simulink model "testmodel"  (R2024b)
settings: Solver=ode23t  StartTime=0.0  StopTime=10  FixedStep=0.0001  MaxStep=0.2  MinStep=0.0001  RelTol=1e-3
model workspace (MAT data in the model file):
  L = 0.57
  La = 0.000279
  Ra = 0.288
  ahead = 0.75
  d = 0.74
  maxrpm = 6000
  pathx : Simulink.Parameter (value not decoded)
  pathy : Simulink.Parameter (value not decoded)
  rover_accel = 0.5
  roveracc = 0.5
  stepangle = 1.8
  w_r = 0.1
  wheelbase = 1
symbols that are objects in the model workspace (value not decoded): pathx, pathy
undefined symbols (not defined in the file): Discrete, Time
libraries: fl_lib x100, nesl_utility x53, ee_lib x15, slpidlib x5, ctrlSharedLib x3, robotalgslib x1, simulink x1
(part 2 of 3)

== system testmodel/control ==
  pos : Inport
  alpha : Inport  Port=2
  R : Inport  Port=3
  goal : Inport  Port=4
  actspeed : Inport  Port=5
  actang : Inport  Port=6
  Constant1 : Constant  Value=d*0.5
  Constant7 : Constant  Value=L
  Mux1 : Mux  Inputs=6
  PID Controller : slpidlib/PID Controller  Controller=PID  Form=Parallel  TimeDomain=Discrete-time  UseExternalTs=off  SampleTime=-1  IntegratorMethod=Forward Euler  FilterMethod=Forward Euler  ControllerParametersSource=internal  P=54.7409706092039  I=0.00122680114575866  UseKiTs=on  D=0.198895104349163  UseExternalDerivativeSource=off  N=8689.11352061538  UseFilter=on  TunerSelectOption=Transfer Function Based (PID Tuner App)  InitialConditionSource=internal  InitialConditionForIntegrator=0  InitialConditionForFilter=0  DifferentiatorICPrevScaledInput=0  ExternalReset=none  TrackingMode=off  Kt=1  LimitOutput=off  SatLimitsSource=internal  UpperSaturationLimit=inf  LowerSaturationLimit=-inf  LinearizeAsGain=on  AntiWindupMode=none  Kb=1  LimitIntegrator=off  UpperIntegratorSaturationLimit=inf  LowerIntegratorSaturationLimit=-inf  POutMin=[]  POutMax=[]  IOutMin=[]  IOutMax=[]  DOutMin=[]  DOutMax=[]  NOutMin=[]  NOutMax=[]  SumOutMin=[]  SumOutMax=[]  SaturationOutMin=[]  SaturationOutMax=[]  PParamMin=[]  PParamMax=[]  IParamMin=[]  IParamMax=[]  DParamMin=[]  DParamMax=[]  NParamMin=[]  NParamMax=[]  KbParamMin=[]  KbParamMax=[]  KtParamMin=[]  KtParamMax=[]  KbOutMin=[]  KbOutMax=[]  KtOutMin=[]  KtOutMax=[]  IntegratorOutMin=[]  IntegratorOutMax=[]  FilterOutMin=[]  FilterOutMax=[]  SumI1OutMin=[]  SumI1OutMax=[]  SumI2OutMin=[]  SumI2OutMax=[]  SumI3OutMin=[]  SumI3OutMax=[]  SumI4OutMin=[]  SumI4OutMax=[]  SumDOutMin=[]  SumDOutMax=[]  DifferentiatorOutMin=[]  DifferentiatorOutMax=[]  FilterDiffOutCoefMin=[]  FilterDiffOutCoefMax=[]  ReciprocalOutMin=[]  ReciprocalOutMax=[]  SumDenOutMin=[]  SumDenOutMax=[]  SumNumOutMin=[]  SumNumOutMax=[]  DivideOutMin=[]  DivideOutMax=[]  UdiffTsProdOutMin=[]  UdiffTsProdOutMax=[]  NTsProdOutMin=[]  NTsProdOutMax=[]  UintegralTsProdOutMin=[]  UintegralTsProdOutMax=[]  UngainTsProdOutMin=[]  UngainTsProdOutMax=[]  ClampingZeroOutDataTypeStr=Inherit: Inherit via back propagation  ClampingZeroOutMin=[]  ClampingZeroOutMax=[]  FilterDenConstantOutDataTypeStr=Inherit: Inherit via back propagation  FilterDenConstantOutMin=[]  FilterDenConstantOutMax=[]  PCopyOutDataTypeStr=Inherit: Inherit via back propagation  PCopyOutMin=[]  PCopyOutMax=[]  NCopyOutDataTypeStr=Inherit: Inherit via back propagation  NCopyOutMin=[]  NCopyOutMax=[]  IntegratorContinuousStateAttributes=''  IntegratorStateMustResolveToSignalObject=off  IntegratorRTWStateStorageClass=Auto  FilterContinuousStateAttributes=''  FilterStateMustResolveToSignalObject=off  FilterRTWStateStorageClass=Auto  ParallelPVariant=InternalParameters  IdealPVariant=Disabled  IVariant=InternalParameters  DVariant=InternalParameters  IntegratorVariant=Discrete  SatVariant=Disabled  AWVariant=Passthrough  PCopyVariant=Disabled  TRVariant=Disabled  FdbkBlocksVariant=Forward  IdealPFdbkVariant=Disabled  SatFdbkVariant=Disabled  DerivativeFilterVariant=ForwardEulerFilter  NVariant=InternalParameters  NCopyVariant=Disabled  FilterICVariant=InternalICsFilter  IntegratorICVariant=InternalICs  ExternalResetVariant=Disabled  TRSumVariant=Passthrough  SumFdbkVariant=Disabled  SumVariant=Sum_PID  TsampFilterVariant=InternalTs  TsampNgainVariant=Passthrough  TsampIntegralVariant=Disabled_SignalSpec  ExternalSaturationOutDataTypeStr=Inherit: Same as second input  DerivativeSourceVariant=ErrorSignal  PreIntVariant=InternalPreInt
  Saturation : Saturate  UpperLimit=24  LowerLimit=-24
  Subsystem1 : Subsystem
  Sum : Sum  Inputs=|+-
  Sum1 : Sum  Inputs=|+-
  Unit Delay : UnitDelay  SampleTime=-1  HasFrameUpgradeWarning=on
  desspeed : Outport
  control : Outport  Port=2
  desang : Outport  Port=3
  angerror : Outport  Port=4
  wires:
  Subsystem1/2(wheel_speed_LM) -> Mux1/2
  Mux1/1 -> Sum/1, desspeed/1
  Subsystem1/3(wheel_speed_LB) -> Mux1/3
  actspeed/1 -> Sum/2
  PID Controller/1 -> Unit Delay/1
  Subsystem1/4(wheel_speed_RF) -> Mux1/4
  Sum/1 -> PID Controller/1
  Subsystem1/6(wheel_speed_RB) -> Mux1/6
  Subsystem1/1(wheel_speed_LF) -> Mux1/1
  Unit Delay/1 -> Saturation/1
  Subsystem1/5(wheel_speed_RM) -> Mux1/5
  alpha/1 -> Subsystem1/1(alpha)
  Constant1/1 -> Subsystem1/3(d)
  Constant7/1 -> Subsystem1/2("L ")
  Saturation/1 -> control/1
  R/1 -> Subsystem1/4("R ")
  pos/1 -> Subsystem1/5(pos)
  goal/1 -> Subsystem1/6(goal)
  Subsystem1/7(desang) -> Sum1/1, desang/1
  actang/1 -> Sum1/2
  Sum1/1 -> angerror/1

== system testmodel/driver ==
  bodyangle : Inport
  gpspos : Inport  Port=2
  encoderpos : Inport  Port=3
  angvwheels : Inport  Port=4
  ref : Inport  Port=5
  bodyangle1 : Inport  Port=6
  gpspos1 : Inport  Port=7
  code : Subsystem
  sim : Subsystem
  controlsignal : Outport
  wires:
  bodyangle/1 -> code/1(bodyangle)
  gpspos/1 -> code/2(gpspos)
  encoderpos/1 -> code/3(encoderpos)
  angvwheels/1 -> code/4(angvwheels)
  ref/1 -> code/5(ref)
  code/1(controlsignal) -> controlsignal/1
  bodyangle1/1 -> sim/1(bodyangle1)
  gpspos1/1 -> sim/2(gpspos1)

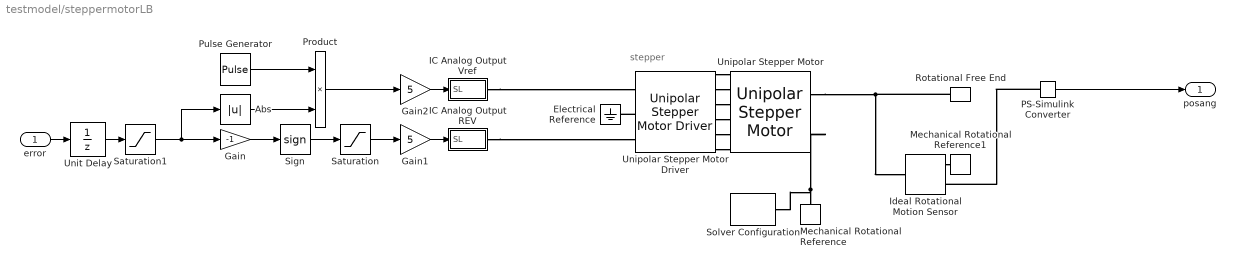
== system testmodel/steppermotorLB ==
  note: stepper
  error : Inport
  Abs : Abs  SaturateOnIntegerOverflow=off
  Electrical Reference : fl_lib/Electrical/Electrical Elements/Electrical Reference
  Gain : Gain  Gain=-1
  Gain1 : Gain  Gain=5
  Gain2 : Gain  Gain=5
  IC Analog Output REV : Subsystem
  IC Analog Output Vref : Subsystem
  Ideal Rotational Motion Sensor : fl_lib/Mechanical/Mechanical Sensors/Ideal Rotational Motion Sensor  reference=foundation.enum.MeasurementReference.difference  acceleration_port=false  velocity_port=false  position_port=true  wrap_angle=false  offset=0 rad
      settings: InternalSimscapePortConfiguration="{\"Bottom\":[],\"Left\":[{\"id\":\"R\",\"label\":\"R\",\"type\":\"foundation.mechanical.rotational.rotational\"}],\"Right\":[{\"id\":\"C\",\"label\":\"C\",\"type\":\"foundation.mechanical.rotational.rotational\"},{\"id\":\"A\",\"label\":\"A\",\"type\":\"output\"}],\"Top\":[]}"
  Mechanical Rotational Reference : fl_lib/Mechanical/Rotational Elements/Mechanical Rotational Reference
  Mechanical Rotational Reference1 : fl_lib/Mechanical/Rotational Elements/Mechanical Rotational Reference
  PS-Simulink Converter : nesl_utility/PS-Simulink Converter  PhysicalDomain=network_engine_domain  SubClassName=ps_output  LeftPortType=input  RightPortType=output  PseudoPeriodic=off  Frequencies=[]  VectorFormat=inherit  Unit=inherit  AffineConversion=off
  Product : Product
  Pulse Generator : DiscretePulseGenerator  Period=10  SampleTime=0.0001
  Rotational Free End : fl_lib/Mechanical/Rotational Elements/Rotational Free End  w_specify=off  w_priority=None  w=0 rad/s  w_nominal_specify=off  w_nominal_value=1  w_nominal_unit=rad/s
  Saturation : Saturate  UpperLimit=1  LowerLimit=0
  Saturation1 : Saturate  UpperLimit=1  LowerLimit=-1
  Sign : Signum
  Solver Configuration : nesl_utility/Solver Configuration  PhysicalDomain=network_engine_domain  SubClassName=solver  LeftPortType=input  RightPortType=generic  Tones=[]  Harmonics=[]  SimulateNoise=off  Profile=off  UseLocalSampling=off  EnableSwitchedLinearOptims=on  FrequencyDomain=off  UseCCode=off  RelTol=0.001  AbsTol=0.001  MinStep=1e-09  ToWorkspace=off  RevertToSquareIcSolve=off  NumHomotopyIterations=100  PhasorMode=off  PhasorModeNumHarmonics=1  ConsistencySolver=NEWTON_XTOL_AFTER_FTOL  IndexReductionMethod=DerivativeReplacement  DoDC=off  ResidualTolerance=1e-09  ConsistencyTolSource=GLOBAL  ConsistencyAbsTol=0.001  ConsistencyRelTol=0.001  ConsistencyTolFactor=0.001  UseLocalSolver=on  LocalSolverChoice=NE_TRAPEZOIDAL_ADVANCER  ResolveIndetEquations=on  FunctionEvalNumThread=1  LocalSolverSampleTime=0.0001  DoFixedCost=off  MaxNonlinIter=3  MaxModeIter=2  ComputeImpulses=off  ImpulseIterations=2  LinearAlgebra=auto  LinearAlgebraNumThread=0  EquationFormulation=NE_TIME_EF  DelaysMemoryBudget=1024  AutomaticFiltering=on  FilteringTimeConstant=0.001  PartitionStorageMethod=AS_NEEDED  PartitionMemoryBudget=1024  PartitionMethod=ROBUST  MultibodyUseLocalSolver=off  MultibodyLocalSolverChoice=ODE1  MultibodyLocalSolverSampleTime=0.001
  Unipolar Stepper Motor : ee_lib/Electromechanical/Reluctance & Stepper/Unipolar Stepper Motor  step_or_av=ee.enum.electromech.simulationMode.stepping  Ra=0.9 Ohm  La=2.2 mH  k=0  Km=0.19 N*m/A  Td=0 N*m  Rm=inf Ohm  w_vec=[0, 1000, 3000] rpm  T_vec=[2, 2, 1] N*m  assert_if_slipping=ee.enum.assertAction.none  J_total=1e-4 kg*m^2  max_step_rate=10 Hz  Step=1.8 deg  J=3.6e-5 kg*m^2  B=8.0e-4 N*m*s/rad  speed0=0 rpm  theta0=0 deg  alpha=3.93e-3 1/K  Tmeas=25 degC  Tmeas2=125 degC  T_vec2=[1.7, 1.7, .85] N*m  half_stepping=ee.enum.electromech.steppingModeAveraged.fullStep  thermal_mass=100 J/K  initial_temperatures=[25, 25, 25, 25] degC  rotor_thermal_mass=50 J/K  rotor_initial_temperature=25 degC  Rm_percent_rotor=90
      settings: InternalSimscapePortConfiguration="{\"Bottom\":[],\"Left\":[{\"id\":\"pA\",\"label\":\"A+\",\"type\":\"foundation.electrical.electrical\"},{\"id\":\"cA\",\"label\":\"A0\",\"type\":\"foundation.electrical.electrical\"},{\"id\":\"nA\",\"label\":\"A-\",\"type\":\"foundation.electrical.electrical\"},{\"id\":\"pB\",\"label\":\"B+\",\"type\":\"foundation.electrical.electrical\"},{\"id\":\"cB\",\"label\":\"B0\",\"type\":\"foundation.electrical.electrical\"},{\"id\":\"nB\",\"label\":\"B-\",\"type\":\"foundation.electrical.electrical\"}],\"Right\":[{\"id\":\"R\",\"label\":\"R\",\"type\":\"foundation.mechanical.rotational.rotational\"},{\"id\":\"C\",\"label\":\"C\",\"type\":\"foundation.mechanical.rotational.rotational\"}],\"Top\":[]}"
  Unipolar Stepper Motor Driver : ee_lib/Electromechanical/Reluctance & Stepper/Unipolar Stepper Motor Driver  step_or_av=ee.enum.electromech.simulationMode.stepping  step_rate_per_volt=10 Hz/V  Venable=0.1 V  Vreverse=0.1 V  Vm=24 V  half_stepping=ee.enum.electromech.steppingModeAveraged.fullStep
      settings: InternalSimscapePortConfiguration="{\"Bottom\":[],\"Left\":[{\"id\":\"ENA\",\"label\":\"ENA\",\"type\":\"foundation.electrical.electrical\"},{\"id\":\"REF\",\"label\":\"REF\",\"type\":\"foundation.electrical.electrical\"},{\"id\":\"REV\",\"label\":\"REV\",\"type\":\"foundation.electrical.electrical\"}],\"Right\":[{\"id\":\"pA\",\"label\":\"A+\",\"type\":\"foundation.electrical.electrical\"},{\"id\":\"cA\",\"label\":\"A0\",\"type\":\"foundation.electrical.electrical\"},{\"id\":\"nA\",\"label\":\"A-\",\"type\":\"foundation.electrical.electrical\"},{\"id\":\"pB\",\"label\":\"B+\",\"type\":\"foundation.electrical.electrical\"},{\"id\":\"cB\",\"label\":\"B0\",\"type\":\"foundation.electrical.electrical\"},{\"id\":\"nB\",\"label\":\"B-\",\"type\":\"foundation.electrical.electrical\"}],\"Top\":[]}"
  Unit Delay : UnitDelay  SampleTime=-1  HasFrameUpgradeWarning=on
  posang : Outport
  wires:
  PS-Simulink Converter/1 -> posang/1
  Gain/1 -> Sign/1
  Sign/1 -> Saturation/1
  Pulse Generator/1 -> Product/1
  Saturation/1 -> Gain1/1
  Product/1 -> Gain2/1
  Gain2/1 -> IC Analog Output Vref/1(SL)
  Gain1/1 -> IC Analog Output REV/1(SL)
  Abs/1 -> Product/2
  Saturation1/1 -> Abs/1, Gain/1
  error/1 -> Unit Delay/1
  Unit Delay/1 -> Saturation1/1
  connections:
  Unipolar Stepper Motor Driver/RConn3 -- Unipolar Stepper Motor/LConn3
  Unipolar Stepper Motor Driver/RConn1 -- Unipolar Stepper Motor/LConn1
  Unipolar Stepper Motor Driver/RConn6 -- Unipolar Stepper Motor/LConn6
  Unipolar Stepper Motor Driver/RConn2 -- Unipolar Stepper Motor/LConn2
  Unipolar Stepper Motor Driver/RConn4 -- Unipolar Stepper Motor/LConn4
  Unipolar Stepper Motor Driver/RConn5 -- Unipolar Stepper Motor/LConn5
  Unipolar Stepper Motor/RConn1 -- Ideal Rotational Motion Sensor/LConn1 -- Rotational Free End/LConn1
  Unipolar Stepper Motor Driver/LConn2 -- Electrical Reference/LConn1
  PS-Simulink Converter/LConn1 -- Ideal Rotational Motion Sensor/RConn2
  Ideal Rotational Motion Sensor/RConn1 -- Mechanical Rotational Reference1/LConn1
  Mechanical Rotational Reference/LConn1 -- Unipolar Stepper Motor/RConn2 -- Solver Configuration/RConn1
  IC Analog Output Vref/RConn1 -- Unipolar Stepper Motor Driver/LConn1
  IC Analog Output REV/RConn1 -- Unipolar Stepper Motor Driver/LConn3

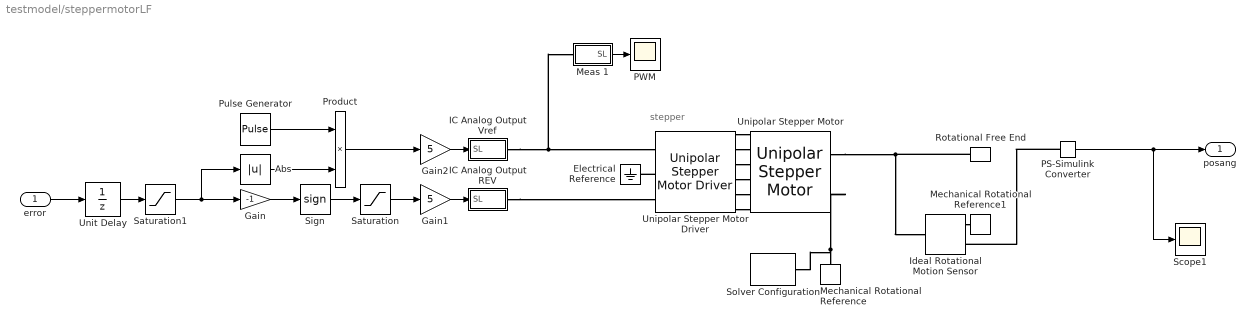
== system testmodel/steppermotorLF ==
  note: stepper
  error : Inport
  Abs : Abs  SaturateOnIntegerOverflow=off
  Electrical Reference : fl_lib/Electrical/Electrical Elements/Electrical Reference
  Gain : Gain  Gain=-1
  Gain1 : Gain  Gain=5
  Gain2 : Gain  Gain=5
  IC Analog Output REV : Subsystem
  IC Analog Output Vref : Subsystem
  Ideal Rotational Motion Sensor : fl_lib/Mechanical/Mechanical Sensors/Ideal Rotational Motion Sensor  reference=foundation.enum.MeasurementReference.difference  acceleration_port=false  velocity_port=false  position_port=true  wrap_angle=false  offset=0 rad
      settings: InternalSimscapePortConfiguration="{\"Bottom\":[],\"Left\":[{\"id\":\"R\",\"label\":\"R\",\"type\":\"foundation.mechanical.rotational.rotational\"}],\"Right\":[{\"id\":\"C\",\"label\":\"C\",\"type\":\"foundation.mechanical.rotational.rotational\"},{\"id\":\"A\",\"label\":\"A\",\"type\":\"output\"}],\"Top\":[]}"
  Meas 1 : Subsystem
  Mechanical Rotational Reference : fl_lib/Mechanical/Rotational Elements/Mechanical Rotational Reference
  Mechanical Rotational Reference1 : fl_lib/Mechanical/Rotational Elements/Mechanical Rotational Reference
  PS-Simulink Converter : nesl_utility/PS-Simulink Converter  PhysicalDomain=network_engine_domain  SubClassName=ps_output  LeftPortType=input  RightPortType=output  PseudoPeriodic=off  Frequencies=[]  VectorFormat=inherit  Unit=inherit  AffineConversion=off
  PWM : Scope
  Product : Product
  Pulse Generator : DiscretePulseGenerator  Period=10  SampleTime=0.0001
  Rotational Free End : fl_lib/Mechanical/Rotational Elements/Rotational Free End  w_specify=off  w_priority=None  w=0 rad/s  w_nominal_specify=off  w_nominal_value=1  w_nominal_unit=rad/s
  Saturation : Saturate  UpperLimit=1  LowerLimit=0
  Saturation1 : Saturate  UpperLimit=1  LowerLimit=-1
  Scope1 : Scope
  Sign : Signum
  Solver Configuration : nesl_utility/Solver Configuration  PhysicalDomain=network_engine_domain  SubClassName=solver  LeftPortType=input  RightPortType=generic  Tones=[]  Harmonics=[]  SimulateNoise=off  Profile=off  UseLocalSampling=off  EnableSwitchedLinearOptims=on  FrequencyDomain=off  UseCCode=off  RelTol=0.001  AbsTol=0.001  MinStep=1e-09  ToWorkspace=off  RevertToSquareIcSolve=off  NumHomotopyIterations=100  PhasorMode=off  PhasorModeNumHarmonics=1  ConsistencySolver=NEWTON_XTOL_AFTER_FTOL  IndexReductionMethod=DerivativeReplacement  DoDC=off  ResidualTolerance=1e-09  ConsistencyTolSource=GLOBAL  ConsistencyAbsTol=0.001  ConsistencyRelTol=0.001  ConsistencyTolFactor=0.001  UseLocalSolver=on  LocalSolverChoice=NE_TRAPEZOIDAL_ADVANCER  ResolveIndetEquations=on  FunctionEvalNumThread=1  LocalSolverSampleTime=0.0001  DoFixedCost=off  MaxNonlinIter=3  MaxModeIter=2  ComputeImpulses=off  ImpulseIterations=2  LinearAlgebra=auto  LinearAlgebraNumThread=0  EquationFormulation=NE_TIME_EF  DelaysMemoryBudget=1024  AutomaticFiltering=on  FilteringTimeConstant=0.001  PartitionStorageMethod=AS_NEEDED  PartitionMemoryBudget=1024  PartitionMethod=ROBUST  MultibodyUseLocalSolver=off  MultibodyLocalSolverChoice=ODE1  MultibodyLocalSolverSampleTime=0.001
  Unipolar Stepper Motor : ee_lib/Electromechanical/Reluctance & Stepper/Unipolar Stepper Motor  step_or_av=ee.enum.electromech.simulationMode.stepping  Ra=0.9 Ohm  La=2.2 mH  k=0  Km=0.19 N*m/A  Td=0 N*m  Rm=inf Ohm  w_vec=[0, 1000, 3000] rpm  T_vec=[2, 2, 1] N*m  assert_if_slipping=ee.enum.assertAction.none  J_total=1e-4 kg*m^2  max_step_rate=10 Hz  Step=1.8 deg  J=3.6e-5 kg*m^2  B=8.0e-4 N*m*s/rad  speed0=0 rpm  theta0=0 deg  alpha=3.93e-3 1/K  Tmeas=25 degC  Tmeas2=125 degC  T_vec2=[1.7, 1.7, .85] N*m  half_stepping=ee.enum.electromech.steppingModeAveraged.fullStep  thermal_mass=100 J/K  initial_temperatures=[25, 25, 25, 25] degC  rotor_thermal_mass=50 J/K  rotor_initial_temperature=25 degC  Rm_percent_rotor=90
      settings: InternalSimscapePortConfiguration="{\"Bottom\":[],\"Left\":[{\"id\":\"pA\",\"label\":\"A+\",\"type\":\"foundation.electrical.electrical\"},{\"id\":\"cA\",\"label\":\"A0\",\"type\":\"foundation.electrical.electrical\"},{\"id\":\"nA\",\"label\":\"A-\",\"type\":\"foundation.electrical.electrical\"},{\"id\":\"pB\",\"label\":\"B+\",\"type\":\"foundation.electrical.electrical\"},{\"id\":\"cB\",\"label\":\"B0\",\"type\":\"foundation.electrical.electrical\"},{\"id\":\"nB\",\"label\":\"B-\",\"type\":\"foundation.electrical.electrical\"}],\"Right\":[{\"id\":\"R\",\"label\":\"R\",\"type\":\"foundation.mechanical.rotational.rotational\"},{\"id\":\"C\",\"label\":\"C\",\"type\":\"foundation.mechanical.rotational.rotational\"}],\"Top\":[]}"
  Unipolar Stepper Motor Driver : ee_lib/Electromechanical/Reluctance & Stepper/Unipolar Stepper Motor Driver  step_or_av=ee.enum.electromech.simulationMode.stepping  step_rate_per_volt=10 Hz/V  Venable=0.1 V  Vreverse=0.1 V  Vm=24 V  half_stepping=ee.enum.electromech.steppingModeAveraged.fullStep
      settings: InternalSimscapePortConfiguration="{\"Bottom\":[],\"Left\":[{\"id\":\"ENA\",\"label\":\"ENA\",\"type\":\"foundation.electrical.electrical\"},{\"id\":\"REF\",\"label\":\"REF\",\"type\":\"foundation.electrical.electrical\"},{\"id\":\"REV\",\"label\":\"REV\",\"type\":\"foundation.electrical.electrical\"}],\"Right\":[{\"id\":\"pA\",\"label\":\"A+\",\"type\":\"foundation.electrical.electrical\"},{\"id\":\"cA\",\"label\":\"A0\",\"type\":\"foundation.electrical.electrical\"},{\"id\":\"nA\",\"label\":\"A-\",\"type\":\"foundation.electrical.electrical\"},{\"id\":\"pB\",\"label\":\"B+\",\"type\":\"foundation.electrical.electrical\"},{\"id\":\"cB\",\"label\":\"B0\",\"type\":\"foundation.electrical.electrical\"},{\"id\":\"nB\",\"label\":\"B-\",\"type\":\"foundation.electrical.electrical\"}],\"Top\":[]}"
  Unit Delay : UnitDelay  SampleTime=-1  HasFrameUpgradeWarning=on
  posang : Outport
  wires:
  PS-Simulink Converter/1 -> Scope1/1, posang/1
  Gain/1 -> Sign/1
  Sign/1 -> Saturation/1
  Pulse Generator/1 -> Product/1
  Saturation/1 -> Gain1/1
  Product/1 -> Gain2/1
  Gain2/1 -> IC Analog Output Vref/1(SL)
  Gain1/1 -> IC Analog Output REV/1(SL)
  Abs/1 -> Product/2
  Meas 1/1(SL) -> PWM/1
  Saturation1/1 -> Abs/1, Gain/1
  error/1 -> Unit Delay/1
  Unit Delay/1 -> Saturation1/1
  connections:
  Unipolar Stepper Motor Driver/RConn3 -- Unipolar Stepper Motor/LConn3
  Unipolar Stepper Motor Driver/RConn1 -- Unipolar Stepper Motor/LConn1
  Unipolar Stepper Motor Driver/RConn6 -- Unipolar Stepper Motor/LConn6
  Unipolar Stepper Motor Driver/RConn2 -- Unipolar Stepper Motor/LConn2
  Unipolar Stepper Motor Driver/RConn4 -- Unipolar Stepper Motor/LConn4
  Unipolar Stepper Motor Driver/RConn5 -- Unipolar Stepper Motor/LConn5
  Unipolar Stepper Motor/RConn1 -- Rotational Free End/LConn1 -- Ideal Rotational Motion Sensor/LConn1
  Unipolar Stepper Motor Driver/LConn2 -- Electrical Reference/LConn1
  PS-Simulink Converter/LConn1 -- Ideal Rotational Motion Sensor/RConn2
  Ideal Rotational Motion Sensor/RConn1 -- Mechanical Rotational Reference1/LConn1
  Unipolar Stepper Motor/RConn2 -- Solver Configuration/RConn1 -- Mechanical Rotational Reference/LConn1
  IC Analog Output Vref/RConn1 -- Meas 1/LConn1 -- Unipolar Stepper Motor Driver/LConn1
  IC Analog Output REV/RConn1 -- Unipolar Stepper Motor Driver/LConn3

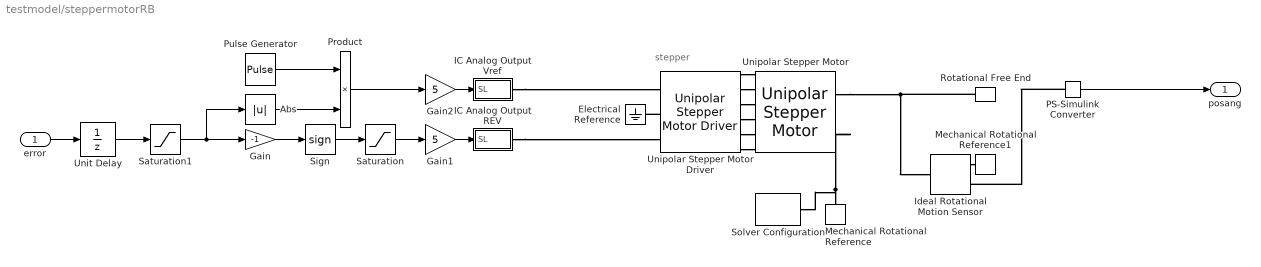
== system testmodel/steppermotorRB ==
  note: stepper
  error : Inport
  Abs : Abs  SaturateOnIntegerOverflow=off
  Electrical Reference : fl_lib/Electrical/Electrical Elements/Electrical Reference
  Gain : Gain  Gain=-1
  Gain1 : Gain  Gain=5
  Gain2 : Gain  Gain=5
  IC Analog Output REV : Subsystem
  IC Analog Output Vref : Subsystem
  Ideal Rotational Motion Sensor : fl_lib/Mechanical/Mechanical Sensors/Ideal Rotational Motion Sensor  reference=foundation.enum.MeasurementReference.difference  acceleration_port=false  velocity_port=false  position_port=true  wrap_angle=false  offset=0 rad
      settings: InternalSimscapePortConfiguration="{\"Bottom\":[],\"Left\":[{\"id\":\"R\",\"label\":\"R\",\"type\":\"foundation.mechanical.rotational.rotational\"}],\"Right\":[{\"id\":\"C\",\"label\":\"C\",\"type\":\"foundation.mechanical.rotational.rotational\"},{\"id\":\"A\",\"label\":\"A\",\"type\":\"output\"}],\"Top\":[]}"
  Mechanical Rotational Reference : fl_lib/Mechanical/Rotational Elements/Mechanical Rotational Reference
  Mechanical Rotational Reference1 : fl_lib/Mechanical/Rotational Elements/Mechanical Rotational Reference
  PS-Simulink Converter : nesl_utility/PS-Simulink Converter  PhysicalDomain=network_engine_domain  SubClassName=ps_output  LeftPortType=input  RightPortType=output  PseudoPeriodic=off  Frequencies=[]  VectorFormat=inherit  Unit=inherit  AffineConversion=off
  Product : Product
  Pulse Generator : DiscretePulseGenerator  Period=10  SampleTime=0.0001
  Rotational Free End : fl_lib/Mechanical/Rotational Elements/Rotational Free End  w_specify=off  w_priority=None  w=0 rad/s  w_nominal_specify=off  w_nominal_value=1  w_nominal_unit=rad/s
  Saturation : Saturate  UpperLimit=1  LowerLimit=0
  Saturation1 : Saturate  UpperLimit=1  LowerLimit=-1
  Sign : Signum
  Solver Configuration : nesl_utility/Solver Configuration  PhysicalDomain=network_engine_domain  SubClassName=solver  LeftPortType=input  RightPortType=generic  Tones=[]  Harmonics=[]  SimulateNoise=off  Profile=off  UseLocalSampling=off  EnableSwitchedLinearOptims=on  FrequencyDomain=off  UseCCode=off  RelTol=0.001  AbsTol=0.001  MinStep=1e-09  ToWorkspace=off  RevertToSquareIcSolve=off  NumHomotopyIterations=100  PhasorMode=off  PhasorModeNumHarmonics=1  ConsistencySolver=NEWTON_XTOL_AFTER_FTOL  IndexReductionMethod=DerivativeReplacement  DoDC=off  ResidualTolerance=1e-09  ConsistencyTolSource=GLOBAL  ConsistencyAbsTol=0.001  ConsistencyRelTol=0.001  ConsistencyTolFactor=0.001  UseLocalSolver=on  LocalSolverChoice=NE_TRAPEZOIDAL_ADVANCER  ResolveIndetEquations=on  FunctionEvalNumThread=1  LocalSolverSampleTime=0.0001  DoFixedCost=off  MaxNonlinIter=3  MaxModeIter=2  ComputeImpulses=off  ImpulseIterations=2  LinearAlgebra=auto  LinearAlgebraNumThread=0  EquationFormulation=NE_TIME_EF  DelaysMemoryBudget=1024  AutomaticFiltering=on  FilteringTimeConstant=0.001  PartitionStorageMethod=AS_NEEDED  PartitionMemoryBudget=1024  PartitionMethod=ROBUST  MultibodyUseLocalSolver=off  MultibodyLocalSolverChoice=ODE1  MultibodyLocalSolverSampleTime=0.001
  Unipolar Stepper Motor : ee_lib/Electromechanical/Reluctance & Stepper/Unipolar Stepper Motor  step_or_av=ee.enum.electromech.simulationMode.stepping  Ra=0.9 Ohm  La=2.2 mH  k=0  Km=0.19 N*m/A  Td=0 N*m  Rm=inf Ohm  w_vec=[0, 1000, 3000] rpm  T_vec=[2, 2, 1] N*m  assert_if_slipping=ee.enum.assertAction.none  J_total=1e-4 kg*m^2  max_step_rate=10 Hz  Step=1.8 deg  J=3.6e-5 kg*m^2  B=8.0e-4 N*m*s/rad  speed0=0 rpm  theta0=0 deg  alpha=3.93e-3 1/K  Tmeas=25 degC  Tmeas2=125 degC  T_vec2=[1.7, 1.7, .85] N*m  half_stepping=ee.enum.electromech.steppingModeAveraged.fullStep  thermal_mass=100 J/K  initial_temperatures=[25, 25, 25, 25] degC  rotor_thermal_mass=50 J/K  rotor_initial_temperature=25 degC  Rm_percent_rotor=90
      settings: InternalSimscapePortConfiguration="{\"Bottom\":[],\"Left\":[{\"id\":\"pA\",\"label\":\"A+\",\"type\":\"foundation.electrical.electrical\"},{\"id\":\"cA\",\"label\":\"A0\",\"type\":\"foundation.electrical.electrical\"},{\"id\":\"nA\",\"label\":\"A-\",\"type\":\"foundation.electrical.electrical\"},{\"id\":\"pB\",\"label\":\"B+\",\"type\":\"foundation.electrical.electrical\"},{\"id\":\"cB\",\"label\":\"B0\",\"type\":\"foundation.electrical.electrical\"},{\"id\":\"nB\",\"label\":\"B-\",\"type\":\"foundation.electrical.electrical\"}],\"Right\":[{\"id\":\"R\",\"label\":\"R\",\"type\":\"foundation.mechanical.rotational.rotational\"},{\"id\":\"C\",\"label\":\"C\",\"type\":\"foundation.mechanical.rotational.rotational\"}],\"Top\":[]}"
  Unipolar Stepper Motor Driver : ee_lib/Electromechanical/Reluctance & Stepper/Unipolar Stepper Motor Driver  step_or_av=ee.enum.electromech.simulationMode.stepping  step_rate_per_volt=10 Hz/V  Venable=0.1 V  Vreverse=0.1 V  Vm=24 V  half_stepping=ee.enum.electromech.steppingModeAveraged.fullStep
      settings: InternalSimscapePortConfiguration="{\"Bottom\":[],\"Left\":[{\"id\":\"ENA\",\"label\":\"ENA\",\"type\":\"foundation.electrical.electrical\"},{\"id\":\"REF\",\"label\":\"REF\",\"type\":\"foundation.electrical.electrical\"},{\"id\":\"REV\",\"label\":\"REV\",\"type\":\"foundation.electrical.electrical\"}],\"Right\":[{\"id\":\"pA\",\"label\":\"A+\",\"type\":\"foundation.electrical.electrical\"},{\"id\":\"cA\",\"label\":\"A0\",\"type\":\"foundation.electrical.electrical\"},{\"id\":\"nA\",\"label\":\"A-\",\"type\":\"foundation.electrical.electrical\"},{\"id\":\"pB\",\"label\":\"B+\",\"type\":\"foundation.electrical.electrical\"},{\"id\":\"cB\",\"label\":\"B0\",\"type\":\"foundation.electrical.electrical\"},{\"id\":\"nB\",\"label\":\"B-\",\"type\":\"foundation.electrical.electrical\"}],\"Top\":[]}"
  Unit Delay : UnitDelay  SampleTime=-1  HasFrameUpgradeWarning=on
  posang : Outport
  wires:
  PS-Simulink Converter/1 -> posang/1
  Gain/1 -> Sign/1
  Sign/1 -> Saturation/1
  Pulse Generator/1 -> Product/1
  Saturation/1 -> Gain1/1
  Product/1 -> Gain2/1
  Gain2/1 -> IC Analog Output Vref/1(SL)
  Gain1/1 -> IC Analog Output REV/1(SL)
  Abs/1 -> Product/2
  Saturation1/1 -> Abs/1, Gain/1
  error/1 -> Unit Delay/1
  Unit Delay/1 -> Saturation1/1
  connections:
  Unipolar Stepper Motor Driver/RConn3 -- Unipolar Stepper Motor/LConn3
  Unipolar Stepper Motor Driver/RConn1 -- Unipolar Stepper Motor/LConn1
  Unipolar Stepper Motor Driver/RConn6 -- Unipolar Stepper Motor/LConn6
  Unipolar Stepper Motor Driver/RConn2 -- Unipolar Stepper Motor/LConn2
  Unipolar Stepper Motor Driver/RConn4 -- Unipolar Stepper Motor/LConn4
  Unipolar Stepper Motor Driver/RConn5 -- Unipolar Stepper Motor/LConn5
  Unipolar Stepper Motor/RConn1 -- Ideal Rotational Motion Sensor/LConn1 -- Rotational Free End/LConn1
  Unipolar Stepper Motor Driver/LConn2 -- Electrical Reference/LConn1
  PS-Simulink Converter/LConn1 -- Ideal Rotational Motion Sensor/RConn2
  Ideal Rotational Motion Sensor/RConn1 -- Mechanical Rotational Reference1/LConn1
  Mechanical Rotational Reference/LConn1 -- Unipolar Stepper Motor/RConn2 -- Solver Configuration/RConn1
  IC Analog Output Vref/RConn1 -- Unipolar Stepper Motor Driver/LConn1
  IC Analog Output REV/RConn1 -- Unipolar Stepper Motor Driver/LConn3

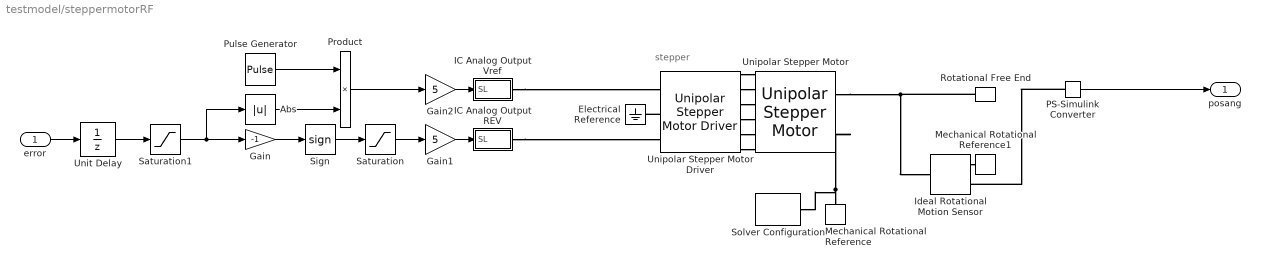
== system testmodel/steppermotorRF ==
  note: stepper
  error : Inport
  Abs : Abs  SaturateOnIntegerOverflow=off
  Electrical Reference : fl_lib/Electrical/Electrical Elements/Electrical Reference
  Gain : Gain  Gain=-1
  Gain1 : Gain  Gain=5
  Gain2 : Gain  Gain=5
  IC Analog Output REV : Subsystem
  IC Analog Output Vref : Subsystem
  Ideal Rotational Motion Sensor : fl_lib/Mechanical/Mechanical Sensors/Ideal Rotational Motion Sensor  reference=foundation.enum.MeasurementReference.difference  acceleration_port=false  velocity_port=false  position_port=true  wrap_angle=false  offset=0 rad
      settings: InternalSimscapePortConfiguration="{\"Bottom\":[],\"Left\":[{\"id\":\"R\",\"label\":\"R\",\"type\":\"foundation.mechanical.rotational.rotational\"}],\"Right\":[{\"id\":\"C\",\"label\":\"C\",\"type\":\"foundation.mechanical.rotational.rotational\"},{\"id\":\"A\",\"label\":\"A\",\"type\":\"output\"}],\"Top\":[]}"
  Mechanical Rotational Reference : fl_lib/Mechanical/Rotational Elements/Mechanical Rotational Reference
  Mechanical Rotational Reference1 : fl_lib/Mechanical/Rotational Elements/Mechanical Rotational Reference
  PS-Simulink Converter : nesl_utility/PS-Simulink Converter  PhysicalDomain=network_engine_domain  SubClassName=ps_output  LeftPortType=input  RightPortType=output  PseudoPeriodic=off  Frequencies=[]  VectorFormat=inherit  Unit=inherit  AffineConversion=off
  Product : Product
  Pulse Generator : DiscretePulseGenerator  Period=10  SampleTime=0.0001
  Rotational Free End : fl_lib/Mechanical/Rotational Elements/Rotational Free End  w_specify=off  w_priority=None  w=0 rad/s  w_nominal_specify=off  w_nominal_value=1  w_nominal_unit=rad/s
  Saturation : Saturate  UpperLimit=1  LowerLimit=0
  Saturation1 : Saturate  UpperLimit=1  LowerLimit=-1
  Sign : Signum
  Solver Configuration : nesl_utility/Solver Configuration  PhysicalDomain=network_engine_domain  SubClassName=solver  LeftPortType=input  RightPortType=generic  Tones=[]  Harmonics=[]  SimulateNoise=off  Profile=off  UseLocalSampling=off  EnableSwitchedLinearOptims=on  FrequencyDomain=off  UseCCode=off  RelTol=0.001  AbsTol=0.001  MinStep=1e-09  ToWorkspace=off  RevertToSquareIcSolve=off  NumHomotopyIterations=100  PhasorMode=off  PhasorModeNumHarmonics=1  ConsistencySolver=NEWTON_XTOL_AFTER_FTOL  IndexReductionMethod=DerivativeReplacement  DoDC=off  ResidualTolerance=1e-09  ConsistencyTolSource=GLOBAL  ConsistencyAbsTol=0.001  ConsistencyRelTol=0.001  ConsistencyTolFactor=0.001  UseLocalSolver=on  LocalSolverChoice=NE_TRAPEZOIDAL_ADVANCER  ResolveIndetEquations=on  FunctionEvalNumThread=1  LocalSolverSampleTime=0.0001  DoFixedCost=off  MaxNonlinIter=3  MaxModeIter=2  ComputeImpulses=off  ImpulseIterations=2  LinearAlgebra=auto  LinearAlgebraNumThread=0  EquationFormulation=NE_TIME_EF  DelaysMemoryBudget=1024  AutomaticFiltering=on  FilteringTimeConstant=0.001  PartitionStorageMethod=AS_NEEDED  PartitionMemoryBudget=1024  PartitionMethod=ROBUST  MultibodyUseLocalSolver=off  MultibodyLocalSolverChoice=ODE1  MultibodyLocalSolverSampleTime=0.001
  Unipolar Stepper Motor : ee_lib/Electromechanical/Reluctance & Stepper/Unipolar Stepper Motor  step_or_av=ee.enum.electromech.simulationMode.stepping  Ra=0.9 Ohm  La=2.2 mH  k=0  Km=0.19 N*m/A  Td=0 N*m  Rm=inf Ohm  w_vec=[0, 1000, 3000] rpm  T_vec=[2, 2, 1] N*m  assert_if_slipping=ee.enum.assertAction.none  J_total=1e-4 kg*m^2  max_step_rate=10 Hz  Step=1.8 deg  J=3.6e-5 kg*m^2  B=8.0e-4 N*m*s/rad  speed0=0 rpm  theta0=0 deg  alpha=3.93e-3 1/K  Tmeas=25 degC  Tmeas2=125 degC  T_vec2=[1.7, 1.7, .85] N*m  half_stepping=ee.enum.electromech.steppingModeAveraged.fullStep  thermal_mass=100 J/K  initial_temperatures=[25, 25, 25, 25] degC  rotor_thermal_mass=50 J/K  rotor_initial_temperature=25 degC  Rm_percent_rotor=90
      settings: InternalSimscapePortConfiguration="{\"Bottom\":[],\"Left\":[{\"id\":\"pA\",\"label\":\"A+\",\"type\":\"foundation.electrical.electrical\"},{\"id\":\"cA\",\"label\":\"A0\",\"type\":\"foundation.electrical.electrical\"},{\"id\":\"nA\",\"label\":\"A-\",\"type\":\"foundation.electrical.electrical\"},{\"id\":\"pB\",\"label\":\"B+\",\"type\":\"foundation.electrical.electrical\"},{\"id\":\"cB\",\"label\":\"B0\",\"type\":\"foundation.electrical.electrical\"},{\"id\":\"nB\",\"label\":\"B-\",\"type\":\"foundation.electrical.electrical\"}],\"Right\":[{\"id\":\"R\",\"label\":\"R\",\"type\":\"foundation.mechanical.rotational.rotational\"},{\"id\":\"C\",\"label\":\"C\",\"type\":\"foundation.mechanical.rotational.rotational\"}],\"Top\":[]}"
  Unipolar Stepper Motor Driver : ee_lib/Electromechanical/Reluctance & Stepper/Unipolar Stepper Motor Driver  step_or_av=ee.enum.electromech.simulationMode.stepping  step_rate_per_volt=10 Hz/V  Venable=0.1 V  Vreverse=0.1 V  Vm=24 V  half_stepping=ee.enum.electromech.steppingModeAveraged.fullStep
      settings: InternalSimscapePortConfiguration="{\"Bottom\":[],\"Left\":[{\"id\":\"ENA\",\"label\":\"ENA\",\"type\":\"foundation.electrical.electrical\"},{\"id\":\"REF\",\"label\":\"REF\",\"type\":\"foundation.electrical.electrical\"},{\"id\":\"REV\",\"label\":\"REV\",\"type\":\"foundation.electrical.electrical\"}],\"Right\":[{\"id\":\"pA\",\"label\":\"A+\",\"type\":\"foundation.electrical.electrical\"},{\"id\":\"cA\",\"label\":\"A0\",\"type\":\"foundation.electrical.electrical\"},{\"id\":\"nA\",\"label\":\"A-\",\"type\":\"foundation.electrical.electrical\"},{\"id\":\"pB\",\"label\":\"B+\",\"type\":\"foundation.electrical.electrical\"},{\"id\":\"cB\",\"label\":\"B0\",\"type\":\"foundation.electrical.electrical\"},{\"id\":\"nB\",\"label\":\"B-\",\"type\":\"foundation.electrical.electrical\"}],\"Top\":[]}"
  Unit Delay : UnitDelay  SampleTime=-1  HasFrameUpgradeWarning=on
  posang : Outport
  wires:
  PS-Simulink Converter/1 -> posang/1
  Gain/1 -> Sign/1
  Sign/1 -> Saturation/1
  Pulse Generator/1 -> Product/1
  Saturation/1 -> Gain1/1
  Product/1 -> Gain2/1
  Gain2/1 -> IC Analog Output Vref/1(SL)
  Gain1/1 -> IC Analog Output REV/1(SL)
  Abs/1 -> Product/2
  Saturation1/1 -> Abs/1, Gain/1
  error/1 -> Unit Delay/1
  Unit Delay/1 -> Saturation1/1
  connections:
  Unipolar Stepper Motor Driver/RConn3 -- Unipolar Stepper Motor/LConn3
  Unipolar Stepper Motor Driver/RConn1 -- Unipolar Stepper Motor/LConn1
  Unipolar Stepper Motor Driver/RConn6 -- Unipolar Stepper Motor/LConn6
  Unipolar Stepper Motor Driver/RConn2 -- Unipolar Stepper Motor/LConn2
  Unipolar Stepper Motor Driver/RConn4 -- Unipolar Stepper Motor/LConn4
  Unipolar Stepper Motor Driver/RConn5 -- Unipolar Stepper Motor/LConn5
  Unipolar Stepper Motor/RConn1 -- Ideal Rotational Motion Sensor/LConn1 -- Rotational Free End/LConn1
  Unipolar Stepper Motor Driver/LConn2 -- Electrical Reference/LConn1
  PS-Simulink Converter/LConn1 -- Ideal Rotational Motion Sensor/RConn2
  Ideal Rotational Motion Sensor/RConn1 -- Mechanical Rotational Reference1/LConn1
  Mechanical Rotational Reference/LConn1 -- Unipolar Stepper Motor/RConn2 -- Solver Configuration/RConn1
  IC Analog Output Vref/RConn1 -- Unipolar Stepper Motor Driver/LConn1
  IC Analog Output REV/RConn1 -- Unipolar Stepper Motor Driver/LConn3

== system testmodel/Path Planning and Navigation WIP/Subsystem1 ==
  tdir : Inport
  Atan : Trigonometry  Operator=atan
  Gain : Gain  Gain=(2*wheelbase)/ahead
  Sine Wave : Sin  TimeSource=Use external signal  SampleTime=0
  rad2deg : Gain  Gain=180/pi
  steerang : Outport
  wires:
  Sine Wave/1 -> Gain/1
  rad2deg/1 -> steerang/1
  Gain/1 -> Atan/1
  Atan/1 -> rad2deg/1
  tdir/1 -> Sine Wave/1

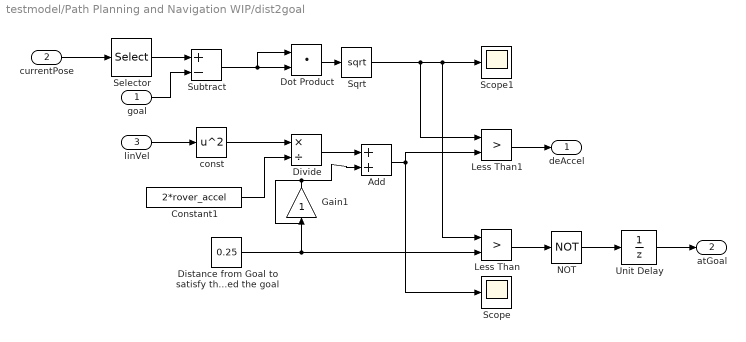
== system testmodel/Path Planning and Navigation WIP/dist2goal ==
  goal : Inport
  currentPose : Inport  Port=2
  linVel : Inport  Port=3
  Add : Sum
  Constant1 : Constant  Value=2*rover_accel
  Distance from Goal to satisfy that the robot has reached the goal : Constant  Value=0.25
  Divide : Product  Inputs=*/
  Dot Product : DotProduct  OutDataTypeStr=Inherit: Inherit via internal rule
  Gain1 : Gain
  Less Than : RelationalOperator  Operator=>  OutDataTypeStr=boolean  RndMeth=Simplest  InputSameDT=off
  Less Than1 : RelationalOperator  Operator=>  OutDataTypeStr=boolean  RndMeth=Simplest  InputSameDT=off
  NOT : Logic  Operator=NOT  IconShape=distinctive  AllPortsSameDT=off  OutDataTypeStr=boolean
  Scope : Scope
  Scope1 : Scope
  Selector : Selector  InputPortWidth=3  IndexOptions=Index vector (dialog)  Indices=[1 2]  OutputSizes=1
  Sqrt : Sqrt
  Subtract : Sum  Inputs=+-
  Unit Delay : UnitDelay  SampleTime=-1  HasFrameUpgradeWarning=on
  const : Math  Operator=square
  deAccel : Outport
  atGoal : Outport  Port=2
  wires:
  currentPose/1 -> Selector/1
  linVel/1 -> const/1
  Constant1/1 -> Divide/2
  Distance from Goal to satisfy that the robot has reached the goal/1 -> Gain1/1, Less Than/2
  Sqrt/1 -> Less Than1/1, Less Than/1, Scope1/1
  Selector/1 -> Subtract/1
  goal/1 -> Subtract/2
  Divide/1 -> Add/1
  Gain1/1 -> Add/2
  Add/1 -> Scope/1, Less Than1/2
  Less Than1/1 -> deAccel/1
  Less Than/1 -> NOT/1
  NOT/1 -> Unit Delay/1
  Unit Delay/1 -> atGoal/1
  Dot Product/1 -> Sqrt/1
  const/1 -> Divide/1
  Subtract/1 -> Dot Product/1, Dot Product/2

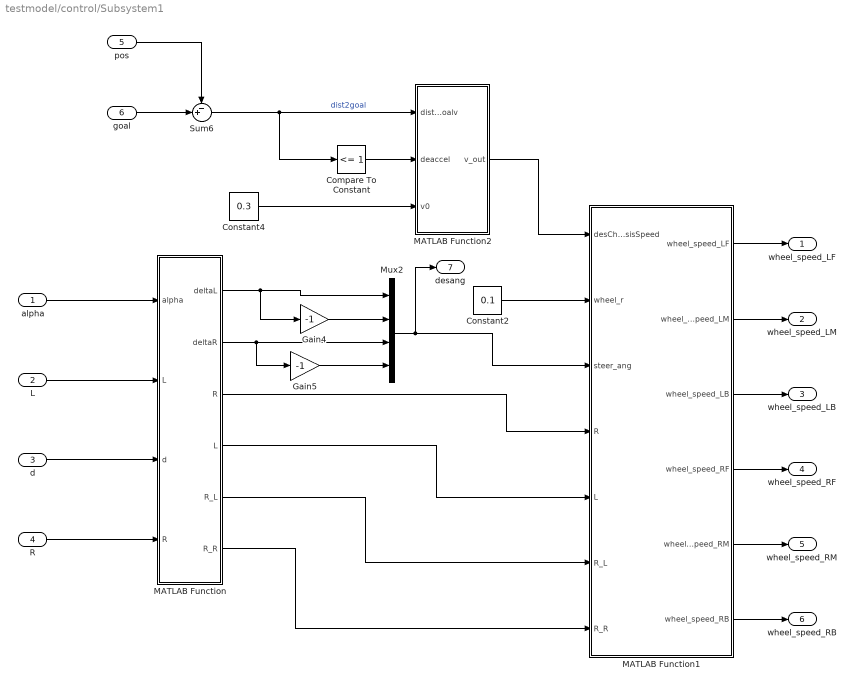
== system testmodel/control/Subsystem1 ==
  alpha : Inport
  "L " : Inport  Port=2
  d : Inport  Port=3
  "R " : Inport  Port=4
  pos : Inport  Port=5
  goal : Inport  Port=6
  Compare To Constant : simulink/Logic and Bit Operations/Compare To Constant  relop=<=  const=1  OutDataTypeStr=boolean
  Constant2 : Constant  Value=0.1
  Constant4 : Constant  Value=0.3
  Gain4 : Gain  Gain=-1
  Gain5 : Gain  Gain=-1
  MATLAB Function : MATLAB Function  TreatAsAtomicUnit=on
  MATLAB Function1 : MATLAB Function  TreatAsAtomicUnit=on
  MATLAB Function2 : MATLAB Function  TreatAsAtomicUnit=on
  Mux2 : Mux
  Sum6 : Sum  Inputs=-+|
  wheel_speed_LF : Outport
  wheel_speed_LM : Outport  Port=2
  wheel_speed_LB : Outport  Port=3
  wheel_speed_RF : Outport  Port=4
  wheel_speed_RM : Outport  Port=5
  wheel_speed_RB : Outport  Port=6
  desang : Outport  Port=7
  wires:
  alpha/1 -> MATLAB Function/1(alpha)
  Constant2/1 -> MATLAB Function1/2(wheel_r)
  MATLAB Function/3(R) -> MATLAB Function1/4(R)
  "R "/1 -> MATLAB Function/4("R ")
  Gain5/1 -> Mux2/4
  MATLAB Function/2(deltaR) -> Gain5/1, Mux2/3
  MATLAB Function/5(R_L) -> MATLAB Function1/6(R_L)
  Gain4/1 -> Mux2/2
  MATLAB Function/4(L) -> MATLAB Function1/5(L)
  MATLAB Function1/6(wheel_speed_RB) -> wheel_speed_RB/1
  MATLAB Function/1(deltaL) -> Gain4/1, Mux2/1
  MATLAB Function/6(R_R) -> MATLAB Function1/7(R_R)
  "L "/1 -> MATLAB Function/2("L ")
  Mux2/1 -> desang/1, MATLAB Function1/3(steer_ang)
  MATLAB Function1/4(wheel_speed_RF) -> wheel_speed_RF/1
  MATLAB Function2/1(v_out) -> MATLAB Function1/1(desChassisSpeed)
  MATLAB Function1/3(wheel_speed_LB) -> wheel_speed_LB/1
  MATLAB Function1/5(wheel_speed_RM) -> wheel_speed_RM/1
  MATLAB Function1/1(wheel_speed_LF) -> wheel_speed_LF/1
  MATLAB Function1/2(wheel_speed_LM) -> wheel_speed_LM/1
  d/1 -> MATLAB Function/3(d)
  Compare To Constant/1 -> MATLAB Function2/2(deaccel)
  Sum6/1 -> MATLAB Function2/1(dist2goalv), Compare To Constant/1  "dist2goal"
  pos/1 -> Sum6/1
  Constant4/1 -> MATLAB Function2/3(v0)
  goal/1 -> Sum6/2

== system testmodel/driver/code ==
  bodyangle : Inport
  gpspos : Inport  Port=2
  encoderpos : Inport  Port=3
  angvwheels : Inport  Port=4
  ref : Inport  Port=5
  Kalman Filter : ctrlSharedLib/Kalman Filter  TimeDomain=Discrete-Time  UseCurrentEstimator=on  ModelSource=LTI State-Space Variable  ModelSourceVariable=ss(1,1,1,0,0.0001)  A=0.95  B=1  C=1  D=0  NumberOfStates=1  NumberOfInputs=1  NumberOfOutputs=1  InitialEstimateSource=Dialog  X0=0  P0=10  UseK=off  UseGH=off  NumberOfProcessNoiseInputs=1  G=1  TimeInvariantG=on  H=0  TimeInvariantH=on  Q=0.05  TimeInvariantQ=on  R=1  TimeInvariantR=on  N=0  TimeInvariantN=on  AddInputPort=on  AddEnablePort=off  OutputEstimatedY=off  OutputP=off  Ts=-1
  PID Controller : slpidlib/PID Controller  Controller=PID  Form=Parallel  TimeDomain=Discrete-time  UseExternalTs=off  SampleTime=0.0001  IntegratorMethod=Forward Euler  FilterMethod=Forward Euler  ControllerParametersSource=internal  P=-14788267.5174  I=-721.927  UseKiTs=on  D=-3770680  UseExternalDerivativeSource=off  N=1577  UseFilter=on  TunerSelectOption=Transfer Function Based (PID Tuner App)  InitialConditionSource=internal  InitialConditionForIntegrator=0  InitialConditionForFilter=0  DifferentiatorICPrevScaledInput=0  ExternalReset=none  TrackingMode=off  Kt=1  LimitOutput=off  SatLimitsSource=internal  UpperSaturationLimit=inf  LowerSaturationLimit=-inf  LinearizeAsGain=on  AntiWindupMode=none  Kb=1  LimitIntegrator=off  UpperIntegratorSaturationLimit=inf  LowerIntegratorSaturationLimit=-inf  POutMin=[]  POutMax=[]  IOutMin=[]  IOutMax=[]  DOutMin=[]  DOutMax=[]  NOutMin=[]  NOutMax=[]  SumOutMin=[]  SumOutMax=[]  SaturationOutMin=[]  SaturationOutMax=[]  PParamMin=[]  PParamMax=[]  IParamMin=[]  IParamMax=[]  DParamMin=[]  DParamMax=[]  NParamMin=[]  NParamMax=[]  KbParamMin=[]  KbParamMax=[]  KtParamMin=[]  KtParamMax=[]  KbOutMin=[]  KbOutMax=[]  KtOutMin=[]  KtOutMax=[]  IntegratorOutMin=[]  IntegratorOutMax=[]  FilterOutMin=[]  FilterOutMax=[]  SumI1OutMin=[]  SumI1OutMax=[]  SumI2OutMin=[]  SumI2OutMax=[]  SumI3OutMin=[]  SumI3OutMax=[]  SumI4OutMin=[]  SumI4OutMax=[]  SumDOutMin=[]  SumDOutMax=[]  DifferentiatorOutMin=[]  DifferentiatorOutMax=[]  FilterDiffOutCoefMin=[]  FilterDiffOutCoefMax=[]  ReciprocalOutMin=[]  ReciprocalOutMax=[]  SumDenOutMin=[]  SumDenOutMax=[]  SumNumOutMin=[]  SumNumOutMax=[]  DivideOutMin=[]  DivideOutMax=[]  UdiffTsProdOutMin=[]  UdiffTsProdOutMax=[]  NTsProdOutMin=[]  NTsProdOutMax=[]  UintegralTsProdOutMin=[]  UintegralTsProdOutMax=[]  UngainTsProdOutMin=[]  UngainTsProdOutMax=[]  ClampingZeroOutDataTypeStr=Inherit: Inherit via back propagation  ClampingZeroOutMin=[]  ClampingZeroOutMax=[]  FilterDenConstantOutDataTypeStr=Inherit: Inherit via back propagation  FilterDenConstantOutMin=[]  FilterDenConstantOutMax=[]  PCopyOutDataTypeStr=Inherit: Inherit via back propagation  PCopyOutMin=[]  PCopyOutMax=[]  NCopyOutDataTypeStr=Inherit: Inherit via back propagation  NCopyOutMin=[]  NCopyOutMax=[]  IntegratorContinuousStateAttributes=''  IntegratorStateMustResolveToSignalObject=off  IntegratorRTWStateStorageClass=Auto  FilterContinuousStateAttributes=''  FilterStateMustResolveToSignalObject=off  FilterRTWStateStorageClass=Auto  ParallelPVariant=InternalParameters  IdealPVariant=Disabled  IVariant=InternalParameters  DVariant=InternalParameters  IntegratorVariant=Discrete  SatVariant=Disabled  AWVariant=Passthrough  PCopyVariant=Disabled  TRVariant=Disabled  FdbkBlocksVariant=Forward  IdealPFdbkVariant=Disabled  SatFdbkVariant=Disabled  DerivativeFilterVariant=ForwardEulerFilter  NVariant=InternalParameters  NCopyVariant=Disabled  FilterICVariant=InternalICsFilter  IntegratorICVariant=InternalICs  ExternalResetVariant=Disabled  TRSumVariant=Passthrough  SumFdbkVariant=Disabled  SumVariant=Sum_PID  TsampFilterVariant=InternalTs  TsampNgainVariant=Passthrough  TsampIntegralVariant=Disabled_SignalSpec  ExternalSaturationOutDataTypeStr=Inherit: Same as second input  DerivativeSourceVariant=ErrorSignal  PreIntVariant=InternalPreInt
  PID Controller1 : slpidlib/PID Controller  Controller=PID  Form=Parallel  TimeDomain=Discrete-time  UseExternalTs=off  SampleTime=0.0001  IntegratorMethod=Forward Euler  FilterMethod=Forward Euler  ControllerParametersSource=internal  P=-5.5999e-07  I=-1.1218e-10  UseKiTs=on  D=2.32908e-10  UseExternalDerivativeSource=off  N=1091  UseFilter=on  TunerSelectOption=Transfer Function Based (PID Tuner App)  InitialConditionSource=internal  InitialConditionForIntegrator=0  InitialConditionForFilter=0  DifferentiatorICPrevScaledInput=0  ExternalReset=none  TrackingMode=off  Kt=1  LimitOutput=off  SatLimitsSource=internal  UpperSaturationLimit=inf  LowerSaturationLimit=-inf  LinearizeAsGain=on  AntiWindupMode=none  Kb=1  LimitIntegrator=off  UpperIntegratorSaturationLimit=inf  LowerIntegratorSaturationLimit=-inf  POutMin=[]  POutMax=[]  IOutMin=[]  IOutMax=[]  DOutMin=[]  DOutMax=[]  NOutMin=[]  NOutMax=[]  SumOutMin=[]  SumOutMax=[]  SaturationOutMin=[]  SaturationOutMax=[]  PParamMin=[]  PParamMax=[]  IParamMin=[]  IParamMax=[]  DParamMin=[]  DParamMax=[]  NParamMin=[]  NParamMax=[]  KbParamMin=[]  KbParamMax=[]  KtParamMin=[]  KtParamMax=[]  KbOutMin=[]  KbOutMax=[]  KtOutMin=[]  KtOutMax=[]  IntegratorOutMin=[]  IntegratorOutMax=[]  FilterOutMin=[]  FilterOutMax=[]  SumI1OutMin=[]  SumI1OutMax=[]  SumI2OutMin=[]  SumI2OutMax=[]  SumI3OutMin=[]  SumI3OutMax=[]  SumI4OutMin=[]  SumI4OutMax=[]  SumDOutMin=[]  SumDOutMax=[]  DifferentiatorOutMin=[]  DifferentiatorOutMax=[]  FilterDiffOutCoefMin=[]  FilterDiffOutCoefMax=[]  ReciprocalOutMin=[]  ReciprocalOutMax=[]  SumDenOutMin=[]  SumDenOutMax=[]  SumNumOutMin=[]  SumNumOutMax=[]  DivideOutMin=[]  DivideOutMax=[]  UdiffTsProdOutMin=[]  UdiffTsProdOutMax=[]  NTsProdOutMin=[]  NTsProdOutMax=[]  UintegralTsProdOutMin=[]  UintegralTsProdOutMax=[]  UngainTsProdOutMin=[]  UngainTsProdOutMax=[]  ClampingZeroOutDataTypeStr=Inherit: Inherit via back propagation  ClampingZeroOutMin=[]  ClampingZeroOutMax=[]  FilterDenConstantOutDataTypeStr=Inherit: Inherit via back propagation  FilterDenConstantOutMin=[]  FilterDenConstantOutMax=[]  PCopyOutDataTypeStr=Inherit: Inherit via back propagation  PCopyOutMin=[]  PCopyOutMax=[]  NCopyOutDataTypeStr=Inherit: Inherit via back propagation  NCopyOutMin=[]  NCopyOutMax=[]  IntegratorContinuousStateAttributes=''  IntegratorStateMustResolveToSignalObject=off  IntegratorRTWStateStorageClass=Auto  FilterContinuousStateAttributes=''  FilterStateMustResolveToSignalObject=off  FilterRTWStateStorageClass=Auto  ParallelPVariant=InternalParameters  IdealPVariant=Disabled  IVariant=InternalParameters  DVariant=InternalParameters  IntegratorVariant=Discrete  SatVariant=Disabled  AWVariant=Passthrough  PCopyVariant=Disabled  TRVariant=Disabled  FdbkBlocksVariant=Forward  IdealPFdbkVariant=Disabled  SatFdbkVariant=Disabled  DerivativeFilterVariant=ForwardEulerFilter  NVariant=InternalParameters  NCopyVariant=Disabled  FilterICVariant=InternalICsFilter  IntegratorICVariant=InternalICs  ExternalResetVariant=Disabled  TRSumVariant=Passthrough  SumFdbkVariant=Disabled  SumVariant=Sum_PID  TsampFilterVariant=InternalTs  TsampNgainVariant=Passthrough  TsampIntegralVariant=Disabled_SignalSpec  ExternalSaturationOutDataTypeStr=Inherit: Same as second input  DerivativeSourceVariant=ErrorSignal  PreIntVariant=InternalPreInt
  Saturation : Saturate  UpperLimit=24  LowerLimit=-24
  Sum : Sum  Inputs=+++
  Sum1 : Sum  Inputs=|+-
  Unit Delay : UnitDelay  SampleTime=-1  HasFrameUpgradeWarning=on
  Unit Delay1 : UnitDelay  SampleTime=-1  HasFrameUpgradeWarning=on
  controlsignal : Outport
  wires:
  bodyangle/1 -> Sum/1
  Sum1/1 -> PID Controller/1
  Saturation/1 -> Unit Delay/1
  PID Controller/1 -> Unit Delay1/1
  Unit Delay1/1 -> Sum/2
  gpspos/1 -> Kalman Filter/1
  ref/1 -> Sum1/1
  Sum/1 -> PID Controller1/1
  PID Controller1/1 -> Saturation/1
  Kalman Filter/1 -> Sum1/2
  encoderpos/1 -> Kalman Filter/2
  Unit Delay/1 -> controlsignal/1
  angvwheels/1 -> Sum/3
